simulink model "two_mass_model_tf"  (R2021b)
settings: Solver=ode8  StartTime=0.0  StopTime=0.25  FixedStep=Tq  RelTol=1e-3
values from neighbouring files (symbols this model uses):
  a0 = a_nom(3)    [calc_params_sensivity.m]    (also in compare_PRs.m; compare_steps.m; neuro_net_testing.m; recalc_training_set.m = acoefs(3))
  a1 = a_nom(2)    [calc_params_sensivity.m]    (also in compare_PRs.m = a_nom(2)*Ttst(2,i); compare_steps.m = a_nom(2)*Ttst(2,vector_num); neuro_net_testing.m = a_nom(2)*Y(2); recalc_training_set.m = acoefs(2))
  a2 = a_nom(1)*Ttst(1,i)    [compare_PRs.m]    (also in compare_steps.m = a_nom(1)*Ttst(1,vector_num); neuro_net_testing.m = a_nom(1)*Y(1); recalc_training_set.m = acoefs(1))
  b0 = b0_v(i)    [calc_params_sensivity.m]    (also in compare_PRs.m = b_nom(1); compare_steps.m = b_nom(1); neuro_net_testing.m = b_nom(1); recalc_training_set.m = bcoefs(1))
  c0 = X(1,1)    [calc_PR.m]    (also in compare_PRs.m = pr_params(1))
  noise_level = 0    [compare_PRs.m]    (also in neuro_net_testing.m; recalc_training_set.m)
  pref_gain = 10*(a_nom(3)*c0/b_nom(1) + r0)    [calc_params_sensivity.m]    (also in compare_PRs.m = 10*(C*c0/Ksp + r0); compare_steps.m; neuro_net_testing.m; test_PR.m = 10*(C*c0/Ksp + r0))
  r0 = X(3,1)    [calc_PR.m]    (also in compare_PRs.m = pr_params(3))
  r1 = X(2,1)    [calc_PR.m]    (also in compare_PRs.m = pr_params(2))
undefined symbols (not defined in the file or in its folder): dec_factor, Tq, Uy
libraries: simulink x1
settings Model: Creator=Ilya  LastModifiedBy=Ilya
settings SolverCC: AlgebraicLoopSolver=TrustRegion
settings DataIOCC: LimitDataPoints=on  SaveFormat=Array  SignalLoggingSaveFormat=ModelDataLogs  ReturnWorkspaceOutputs=off
settings OptimizationCC: BlockReduction=off  BooleanDataType=off  LifeSpan=inf
settings DebuggingCC: SaveWithParameterizedLinksMsg=none  UnderspecifiedInitializationDetection=Classic  MergeDetectMultiDrivingBlocksExec=none  SignalResolutionControl=TryResolveAllWithWarning  MultiTaskDSMMsg=warning  MultiTaskCondExecSysMsg=none  SFUnexpectedBacktrackingDiag=warning  SFNoUnconditionalDefaultTransitionDiag=warning  SFExecutionAtInitializationDiag=none  SFMachineParentedDataDiag=warning  ArithmeticOperatorsInVariantConditions=warning
settings HardwareCC: ProdBitPerPointer=32  ProdBitPerSizeT=32  ProdBitPerPtrDiffT=32  ProdLargestAtomicFloat=None  ProdIntDivRoundTo=Undefined  ProdEndianess=Unspecified  ProdWordSize=32  ProdHWDeviceType=32-bit Generic  TargetUnknown=on
settings ModelReferenceCC: PropagateSignalLabelsOutOfModel=off
settings SFSimCC: SimUseLocalCustomCode=off  CustomCodeUndefinedFunction=UseInterfaceOnly
settings RTWCC: RTWUseLocalCustomCode=off
settings CodeAppCC: StateflowObjectComments=on
settings GRTTargetCC: TargetLangStandard=C89/C90 (ANSI)
settings ConfigComp: CovMetricSettings=dw  CovSaveCumulativeToWorkspaceVar=on  CovSaveSingleToWorkspaceVar=on  CovExternalEMLEnable=off

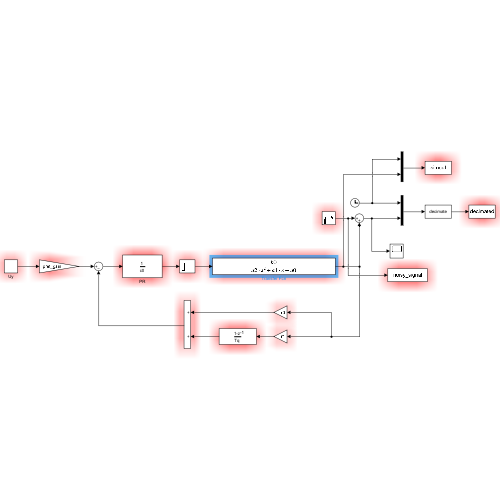
[thumbnail: Simulink's stored preview of the top-level diagram]
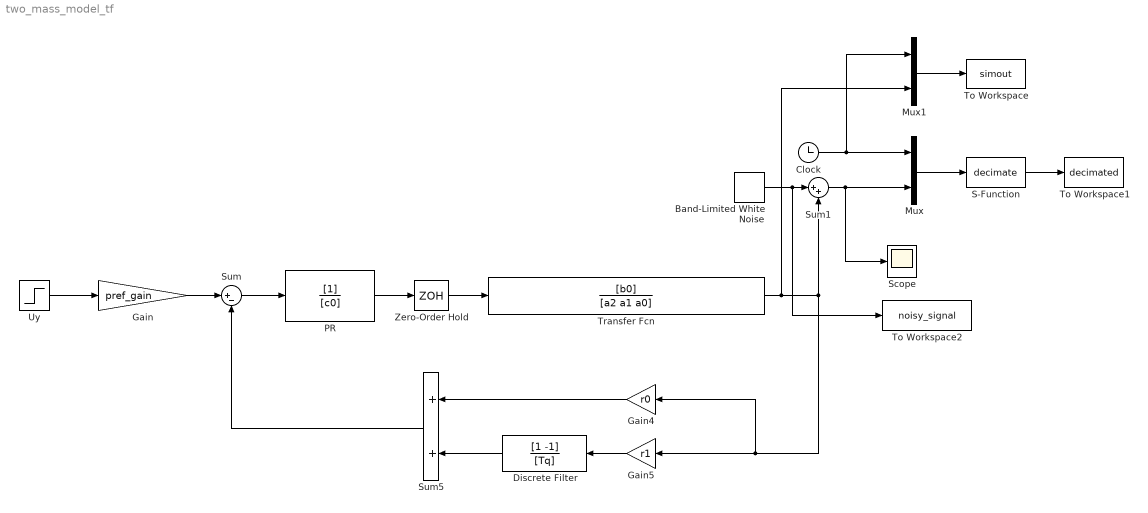
== system two_mass_model_tf ==
  Band-Limited White Noise : simulink/Sources/Band-Limited White Noise  Cov=[noise_level]  Ts=Tq  seed=[23341]
  Clock : Clock
  Discrete Filter : DiscreteFilter  Numerator=[1 -1]  Denominator=[Tq]  SampleTime=Tq
  Gain : Gain  Gain=pref_gain
  Gain4 : Gain  Gain=r0  SampleTime=Tq
  Gain5 : Gain  Gain=r1  SampleTime=Tq
  Mux : Mux  Inputs=2
  Mux1 : Mux  Inputs=2
  PR : DiscreteFilter  Denominator=[c0]  SampleTime=Tq
  S-Function : S-Function  FunctionName=decimate  Parameters=Tq,dec_factor,Uy  SFunctionDeploymentMode=off  EnableBusSupport=off
  Scope : Scope
  Sum : Sum  Inputs=|+-
  Sum1 : Sum  Inputs=|++
  Sum5 : Sum  SampleTime=Tq
  To Workspace : ToWorkspace  VariableName=simout  SampleTime=Tq
  To Workspace1 : ToWorkspace  VariableName=decimated  SampleTime=Tq
      settings: Decimation=dec_factor
  To Workspace2 : ToWorkspace  VariableName=noisy_signal  SampleTime=Tq
  Transfer Fcn : TransferFcn  Numerator=[b0]  Denominator=[a2 a1 a0]
  Uy : Step  Time=0  After=Uy  SampleTime=0
  Zero-Order Hold : ZeroOrderHold  SampleTime=Tq
  wires:
  Uy/1 -> Gain/1
  Gain/1 -> Sum/1
  Sum/1 -> PR/1
  PR/1 -> Zero-Order Hold/1
  Zero-Order Hold/1 -> Transfer Fcn/1
  Transfer Fcn/1 -> Mux1/2, Gain5/1, Gain4/1, Sum1/2
  Gain4/1 -> Sum5/1
  Gain5/1 -> Discrete Filter/1
  Discrete Filter/1 -> Sum5/2
  Sum5/1 -> Sum/2
  Clock/1 -> Mux1/1, Mux/1
  Mux/1 -> S-Function/1
  S-Function/1 -> To Workspace1/1
  Sum1/1 -> Scope/1, Mux/2
  Band-Limited White Noise/1 -> To Workspace2/1, Sum1/1
  Mux1/1 -> To Workspace/1
